simulink model "compare"  (R2016a)
settings: Solver=VariableStepAuto  StartTime=0.0  StopTime=50.0  RelTol=1e-3
libraries: simulink x1
settings Model: Creator=shohei  LastModifiedBy=shohei

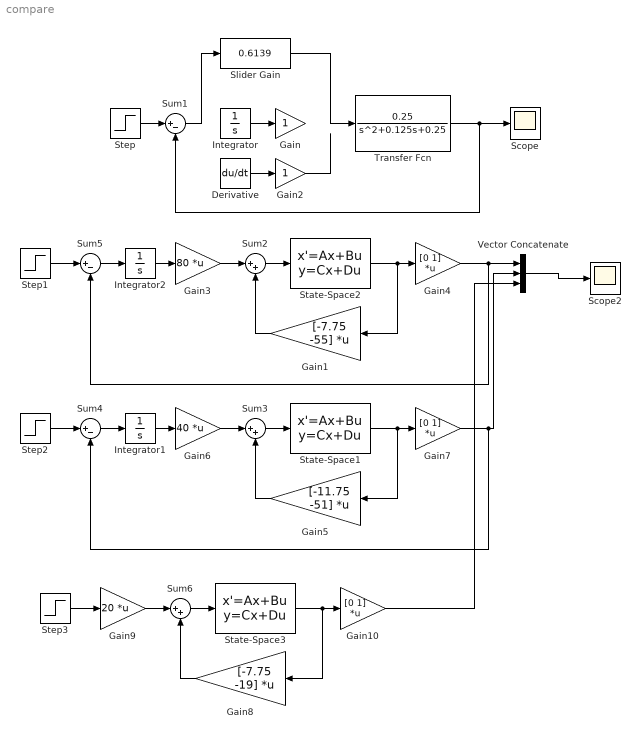
== system compare ==
  Derivative : Derivative
  Gain : Gain
  Gain1 : Gain  Gain=[-7.75 -55]  Multiplication=Matrix(K*u)
  Gain10 : Gain  Gain=[0 1]  Multiplication=Matrix(K*u)
  Gain2 : Gain
  Gain3 : Gain  Gain=80  Multiplication=Matrix(K*u)
  Gain4 : Gain  Gain=[0 1]  Multiplication=Matrix(K*u)
  Gain5 : Gain  Gain=[-11.75 -51]  Multiplication=Matrix(K*u)
  Gain6 : Gain  Gain=40  Multiplication=Matrix(K*u)
  Gain7 : Gain  Gain=[0 1]  Multiplication=Matrix(K*u)
  Gain8 : Gain  Gain=[-7.75 -19]  Multiplication=Matrix(K*u)
  Gain9 : Gain  Gain=20  Multiplication=Matrix(K*u)
  Integrator : Integrator
  Integrator1 : Integrator
  Integrator2 : Integrator
  Scope : Scope
  Scope2 : Scope
  Slider Gain : simulink/Math Operations/Slider Gain  low=0.01  gain=0.6139  high=1
  State-Space1 : StateSpace  A=[-0.125 -0.5; 0.5 0]  B=[0.5;0]  C=eye(2)  D=[0;0]  X0=0
  State-Space2 : StateSpace  A=[-0.125 -0.5; 0.5 0]  B=[0.5;0]  C=eye(2)  D=[0;0]  X0=0
  State-Space3 : StateSpace  A=[-0.125 -0.5; 0.5 0]  B=[0.5;0]  C=eye(2)  D=[0;0]  X0=0
  Step{,1..3} (4 alike) : Step  SampleTime=0
  Sum1 : Sum  Inputs=|+-
  Sum2 : Sum  Inputs=|++
  Sum3 : Sum  Inputs=|++
  Sum4 : Sum  Inputs=|+-
  Sum5 : Sum  Inputs=|+-
  Sum6 : Sum  Inputs=|++
  Transfer Fcn : TransferFcn  Numerator=[0.25]  Denominator=[1 0.125 0.25]
  Vector Concatenate : Concatenate  NumInputs=3
  wires:
  Transfer Fcn/1 -> Sum1/2, Scope/1
  Integrator/1 -> Gain/1
  Step/1 -> Sum1/1
  Sum1/1 -> Slider Gain/1
  Derivative/1 -> Gain2/1
  Slider Gain/1 -> Transfer Fcn/1
  Gain2/1 -> ?
  Gain5/1 -> Sum3/2
  Sum3/1 -> State-Space1/1
  State-Space1/1 -> Gain5/1, Gain7/1
  Gain7/1 -> Vector Concatenate/2, Sum4/2
  Step2/1 -> Sum4/1
  Sum4/1 -> Integrator1/1
  Integrator1/1 -> Gain6/1
  Gain6/1 -> Sum3/1
  Gain1/1 -> Sum2/2
  Sum2/1 -> State-Space2/1
  State-Space2/1 -> Gain1/1, Gain4/1
  Gain4/1 -> Vector Concatenate/1, Sum5/2
  Step1/1 -> Sum5/1
  Sum5/1 -> Integrator2/1
  Integrator2/1 -> Gain3/1
  Gain3/1 -> Sum2/1
  Vector Concatenate/1 -> Scope2/1
  Gain8/1 -> Sum6/2
  Sum6/1 -> State-Space3/1
  State-Space3/1 -> Gain8/1, Gain10/1
  Gain10/1 -> Vector Concatenate/3
  Gain9/1 -> Sum6/1
  Step3/1 -> Gain9/1
